simulink model "lef_linmod"  (R2021a)
settings: Solver=VariableStepAuto  StartTime=0.0  StopTime=10.0  RelTol=1e-3
undefined symbols (not defined in the file or in its folder): trim_state
settings Model: Creator=johnviljoen  LastModifiedBy=johnviljoen

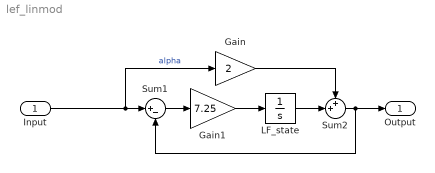
== system lef_linmod ==
  Input : Inport
  Gain : Gain  Gain=2  SaturateOnIntegerOverflow=on  OutDataTypeStr=Inherit: Same as input  ParamDataTypeStr=Inherit: Same as input
  Gain1 : Gain  Gain=7.25  SaturateOnIntegerOverflow=on  OutDataTypeStr=Inherit: Same as input  ParamDataTypeStr=Inherit: Same as input
  LF_state : Integrator  InitialCondition=-trim_state(8)*180/pi
  Sum1 : Sum  Inputs=|+-  InputSameDT=on  SaturateOnIntegerOverflow=on  OutDataTypeStr=Inherit: Same as first input
  Sum2 : Sum  Inputs=++|  InputSameDT=on  SaturateOnIntegerOverflow=on  OutDataTypeStr=Inherit: Same as first input
  Output : Outport
  wires:
  Gain1/1 -> LF_state/1
  Gain/1 -> Sum2/1
  LF_state/1 -> Sum2/2
  Sum1/1 -> Gain1/1
  Sum2/1 -> Output/1, Sum1/2
  Input/1 -> Gain/1, Sum1/1  "alpha"
